simulink model "bras_simulation"  (R2020a)
settings: Solver=VariableStepAuto  StartTime=0.0  StopTime=230  RelTol=1e-3
values from neighbouring files (symbols this model uses):
  a = 10    [bras.m]    (also in bras_espace.m = 43.18; bras_init.m; simulation_couplage_figures.m = plot([0 x1], [0 y1], 'b'))
  b = 12    [bras.m]    (also in bras_espace.m = 31.62; bras_init.m; simulation_couplage_figures.m = plot([x1 x2], [y1 y2], 'r'))
  cond_ini = [10; 10; 10; 0]    [bras.m]    (also in bras_espace.m = [10; 10; 10; 30]; bras_init.m = [10; 10; 10; 30]; init_simulation_couplage.m = [-pi/4; pi/4; -pi/4; 0])
libraries: simulink x1
settings Model: Creator=loloche  LastModifiedBy=loloche

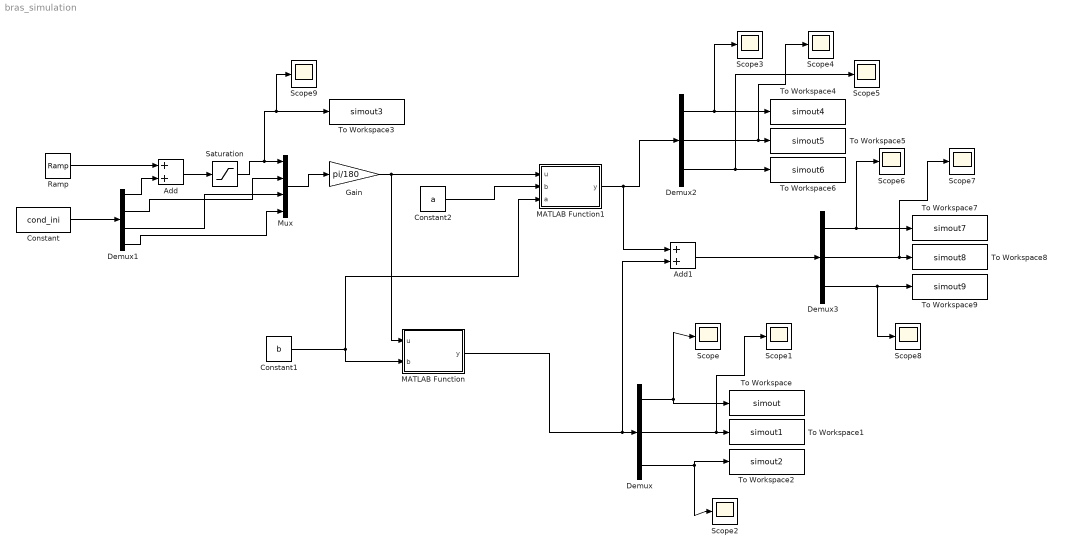
== system bras_simulation ==
  Add : Sum
  Add1 : Sum
  Constant : Constant  Value=cond_ini
  Constant1 : Constant  Value=b
  Constant2 : Constant  Value=a
  Demux : Demux  Outputs=3
  Demux1 : Demux
  Demux2 : Demux  Outputs=3
  Demux3 : Demux  Outputs=3
  Gain : Gain  Gain=pi/180
  MATLAB Function : MATLAB Function  TreatAsAtomicUnit=on
  MATLAB Function1 : MATLAB Function  TreatAsAtomicUnit=on
  Mux : Mux
  Ramp : simulink/Sources/Ramp  slope=1  start=0  InitialOutput=0
  Saturation : Saturate  UpperLimit=240
  Scope{,1..9} (10 alike) : Scope
  To Workspace : ToWorkspace  VariableName=simout  SaveFormat=Structure With Time  SampleTime=-1
  To Workspace1 : ToWorkspace  VariableName=simout1  SaveFormat=Structure With Time  SampleTime=-1
  To Workspace2 : ToWorkspace  VariableName=simout2  SaveFormat=Structure With Time  SampleTime=-1
  To Workspace3 : ToWorkspace  VariableName=simout3  SaveFormat=Structure With Time  SampleTime=-1
  To Workspace4 : ToWorkspace  VariableName=simout4  SaveFormat=Structure With Time  SampleTime=-1
  To Workspace5 : ToWorkspace  VariableName=simout5  SaveFormat=Structure With Time  SampleTime=-1
  To Workspace6 : ToWorkspace  VariableName=simout6  SaveFormat=Structure With Time  SampleTime=-1
  To Workspace7 : ToWorkspace  VariableName=simout7  SaveFormat=Structure With Time  SampleTime=-1
  To Workspace8 : ToWorkspace  VariableName=simout8  SaveFormat=Structure With Time  SampleTime=-1
  To Workspace9 : ToWorkspace  VariableName=simout9  SaveFormat=Structure With Time  SampleTime=-1
  wires:
  Constant1/1 -> MATLAB Function1/3(a), MATLAB Function/2(b)
  MATLAB Function/1(y) -> Add1/2, Demux/1
  Demux/1 -> Scope/1, To Workspace/1
  Demux/2 -> Scope1/1, To Workspace1/1
  Demux/3 -> Scope2/1, To Workspace2/1
  Gain/1 -> MATLAB Function/1(u), MATLAB Function1/1(u)
  Add/1 -> Saturation/1
  Constant/1 -> Demux1/1
  Demux1/1 -> Add/2
  Ramp/1 -> Add/1
  Demux1/2 -> Mux/2
  Demux1/3 -> Mux/3
  Demux1/4 -> Mux/4
  Saturation/1 -> Scope9/1, To Workspace3/1, Mux/1
  Mux/1 -> Gain/1
  Constant2/1 -> MATLAB Function1/2(b)
  Demux2/2 -> Scope4/1, To Workspace5/1
  MATLAB Function1/1(y) -> Add1/1, Demux2/1
  Demux2/1 -> Scope3/1, To Workspace4/1
  Demux2/3 -> Scope5/1, To Workspace6/1
  Demux3/2 -> Scope7/1, To Workspace8/1
  Add1/1 -> Demux3/1
  Demux3/1 -> Scope6/1, To Workspace7/1
  Demux3/3 -> Scope8/1, To Workspace9/1

== matlab function bras_simulation/MATLAB Function ==
  data: u input; y output; b input
function y = fcn(u, b)
theta_x = u(1);
theta_y = u(2);
theta_z = u(3);
y = [-b*sin(theta_y); b*sin(theta_x)*cos(theta_y); -b*cos(theta_x)*cos(theta_y)];

== matlab function bras_simulation/MATLAB Function1 ==
  data: u input; b input; y output; a input
function y = fcn(u, b, a)
theta_x = u(1);
theta_y = u(2);
theta_z = u(3);
phi = u(4);
axx = -a*cos(phi)*sin(theta_y)-a*sin(phi)*cos(theta_y)*sin(theta_z);
axy = a*cos(phi)*sin(theta_x)*cos(theta_y)+a*sin(phi)*cos(theta_x)*cos(theta_z)-a*sin(phi)*sin(theta_x)*sin(theta_y)*sin(theta_z);
axz = -a*cos(phi)*cos(theta_x)*cos(theta_y)+a*sin(phi)*sin(theta_x)*cos(theta_z)+a*sin(phi)*cos(theta_x)*sin(theta_y)*sin(theta_z);
y = [axx; axy; axz];
